simulink model "Richero280245_Assign2"  (R2024b)
settings: Solver=ode5  StartTime=0.0  StopTime=simTime  FixedStep=fixedStepSize  RelTol=1e-3
settings Model: Creator=carlorichero  LastModifiedBy=carlorichero
settings OptimizationCC: DefaultParameterBehavior=Inlined  EnhancedBackFolding=on  PassReuseOutputArgsAs=Individual arguments  ZeroExternalMemoryAtStartup=off  ZeroInternalMemoryAtStartup=off  OptimizeBlockOrder=speed  DifferentSizesBufferReuse=on  OptimizationCustomize=off  EfficientTunableParamExpr=on
settings DebuggingCC: ParameterTunabilityLossMsg=error  ModelReferenceSymbolNameMessage=none
settings ModelReferenceCC: ModelReferenceMinAlgLoopOccurrences=on
settings SFSimCC: MATLABDynamicMemAlloc=off
settings RTWCC: Description=Embedded Coder  SystemTargetFile=ert.tlc  TemplateMakefile=ert_default_tmf
settings CodeAppCC: ForceParamTrailComments=on  IgnoreCustomStorageClasses=off  OperatorAnnotations=on  SimulinkDataObjDesc=on  SFDataObjDesc=on  InsertBlockDesc=on
settings ERTTargetCC: TargetLangStandard=C99 (ISO)  GenerateSampleERTMain=on  SupportContinuousTime=on  ERTCustomFileTemplate=example_file_process.tlc

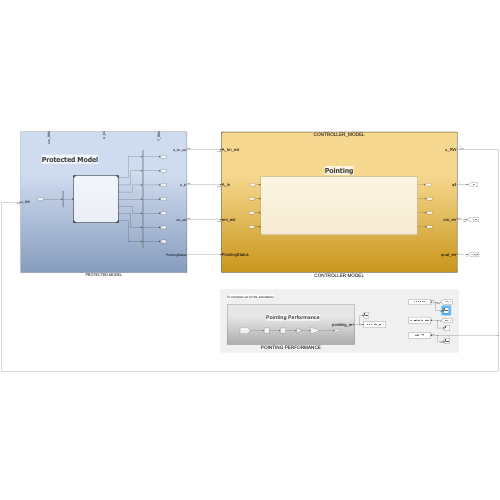
[thumbnail: Simulink's stored preview of the top-level diagram]
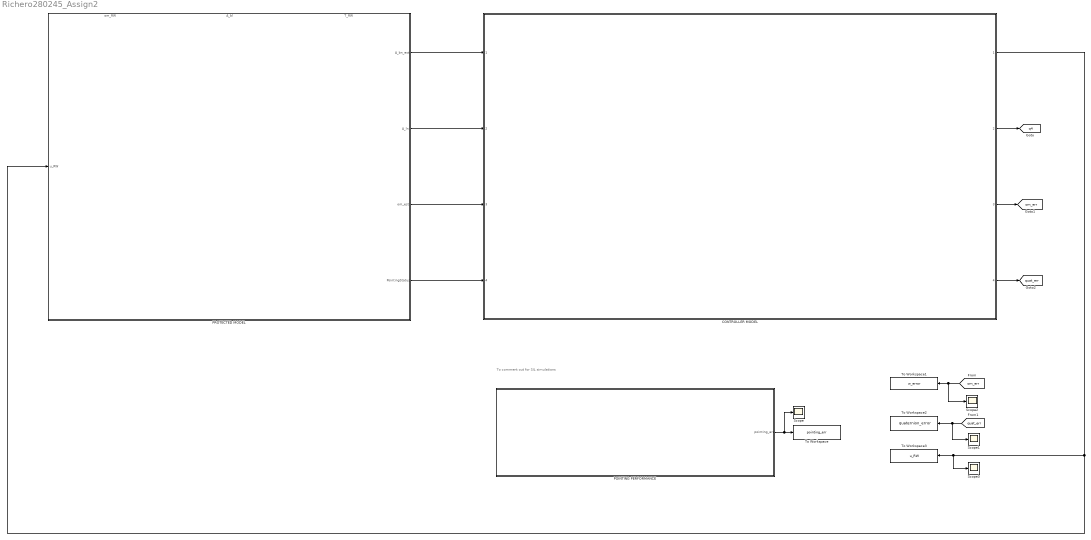
== system Richero280245_Assign2 ==
  note: To comment out for SIL simulations
  CONTROLLER MODEL : Subsystem  TreatAsAtomicUnit=on  ReferencedSubsystem=CONTROLLER_MODEL
  POINTING PERFORMANCE : Subsystem
  PROTECTED MODEL : Subsystem
      settings: PortSchema="{\"entries\":[{\"content\":{\"sides\":[{\"content\":{\"connectorIds\":[\"In1\"]},\"type\":\"ConnectorPlacement.EquallySpacedRectSide\",\"uuid\":\"4269bbd7-3d48-41c9-baab-2de509ebb7e1\"},{\"content\":{\"connectorIds\":[\"Out1\",\"Out2\",\"Out3\",\"Out4\"],\"side\":\"RIGHT\"},\"type\":\"ConnectorPlacement.EquallySpacedRectSide\",\"uuid\":\"222d9627-51e2-4221-8804-06875370038a\"},{\"content\":{\"connectorIds\":[\"Out5\",\"Out6\",\"Out7\"],\"side\":\"TOP\"},\"type\":\"ConnectorPlacement.EquallySpacedRectSide\",\"uuid\":\"776906b1-e520-453d-82b9-997892025e37\"}]},\"type\":\"ConnectorPlacement.EquallySpacedConnector\",\"uuid\":\"d946510d-fad0-4a3e-8089-90c78bf4e7fd\"}],\"packageUris\":[\"http://schema.mathworks.com/mf0/Connector/R2020b\"],\"version\":\"1.0\"}"
  Scope{,1..3} (4 alike) : Scope
  To Workspace : ToWorkspace  VariableName=pointing_err  SampleTime=-1
      settings: Save2DSignal=2-D array (concatenate along first dimension)
  To Workspace1 : ToWorkspace  VariableName=w_error  SampleTime=-1
  To Workspace2 : ToWorkspace  VariableName=quaternion_error  SampleTime=-1
  To Workspace3 : ToWorkspace  VariableName=u_RW  SampleTime=-1
  tag scope: om_err=global, q4=global, quat_err=global
  wires:
  CONTROLLER MODEL/1 -> PROTECTED MODEL/1(u_RW), Scope3/1, To Workspace3/1
  CONTROLLER MODEL/2 -> [q4]
  PROTECTED MODEL/1(A_bn_est) -> CONTROLLER MODEL/1
  PROTECTED MODEL/2(A_ln) -> CONTROLLER MODEL/2
  PROTECTED MODEL/3(om_est) -> CONTROLLER MODEL/3
  PROTECTED MODEL/4(PointingStatus) -> CONTROLLER MODEL/4
  CONTROLLER MODEL/3 -> [om_err]
  CONTROLLER MODEL/4 -> [quat_err]
  POINTING PERFORMANCE/1(pointing_err) -> Scope/1, To Workspace/1
  [quat_err] -> Scope1/1, To Workspace2/1
  [om_err] -> Scope2/1, To Workspace1/1

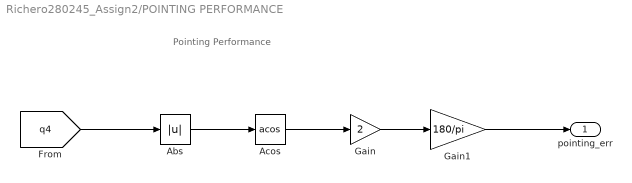
== system Richero280245_Assign2/POINTING PERFORMANCE ==
  note: Pointing Performance
  Abs : Abs  SaturateOnIntegerOverflow=off
  Acos : Trigonometry  Operator=acos
  Gain : Gain  Gain=2
  Gain1 : Gain  Gain=180/pi
  pointing_err : Outport
  wires:
  Acos/1 -> Gain/1
  Abs/1 -> Acos/1
  Gain1/1 -> pointing_err/1
  [q4] -> Abs/1
  Gain/1 -> Gain1/1

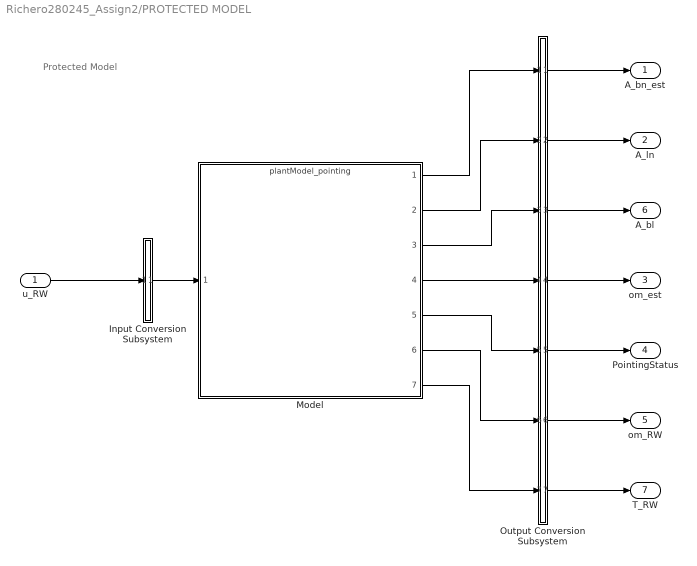
== system Richero280245_Assign2/PROTECTED MODEL ==
  note: Protected Model
  u_RW : Inport
  Input Conversion Subsystem : Subsystem  Tag=__SLT_ICS__  Description=|
      | Signal spec.
      | and routing
      settings: AttributesFormatString=%<Description>
  Model : ModelReference  ModelNameDialog=plantModel_pointing.slxp  ModelReferenceVersion=1.73  CopyOfModelProtected=on
  Output Conversion Subsystem : Subsystem  Tag=__SLT_OCS__  Description=|
      | Signal spec.
      | and routing
      settings: AttributesFormatString=%<Description>
  A_bn_est : Outport
  A_ln : Outport  Port=2
  om_est : Outport  Port=3
  PointingStatus : Outport  Port=4
  om_RW : Outport  Port=5
  A_bl : Outport  Port=6
  T_RW : Outport  Port=7
  wires:
  Model/6 -> Output Conversion Subsystem/6(Inport_6)
  Output Conversion Subsystem/1(Outport_1) -> A_bn_est/1
  Model/2 -> Output Conversion Subsystem/2(Inport_2)
  Output Conversion Subsystem/5(Outport_5) -> PointingStatus/1
  Output Conversion Subsystem/2(Outport_2) -> A_ln/1
  Model/7 -> Output Conversion Subsystem/7(Inport_7)
  Output Conversion Subsystem/7(Outport_7) -> T_RW/1
  Model/1 -> Output Conversion Subsystem/1(Inport_1)
  Model/3 -> Output Conversion Subsystem/3(Inport_3)
  Input Conversion Subsystem/1(Outport_1) -> Model/1
  Model/5 -> Output Conversion Subsystem/5(Inport_5)
  Model/4 -> Output Conversion Subsystem/4(Inport_4)
  Output Conversion Subsystem/6(Outport_6) -> om_RW/1
  Output Conversion Subsystem/4(Outport_4) -> om_est/1
  Output Conversion Subsystem/3(Outport_3) -> A_bl/1
  u_RW/1 -> Input Conversion Subsystem/1(Inport_1)

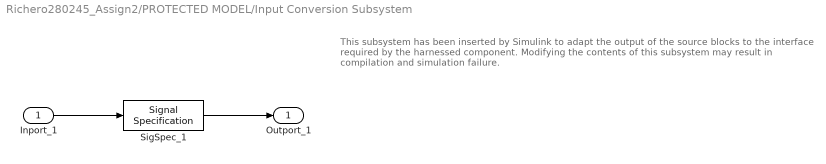
== system Richero280245_Assign2/PROTECTED MODEL/Input Conversion Subsystem ==
  note: This subsystem has been inserted by Simulink to adapt the output of the source blocks to the interface required by the harnessed component.
      |  Modifying the contents of this subsystem may result in compilation and simulation failure.
  Inport_1 : Inport
  SigSpec_1 : SignalSpecification  OutDataTypeStr=double  Dimensions=[3, 1]  SampleTime=0.1
  Outport_1 : Outport
  wires:
  SigSpec_1/1 -> Outport_1/1
  Inport_1/1 -> SigSpec_1/1

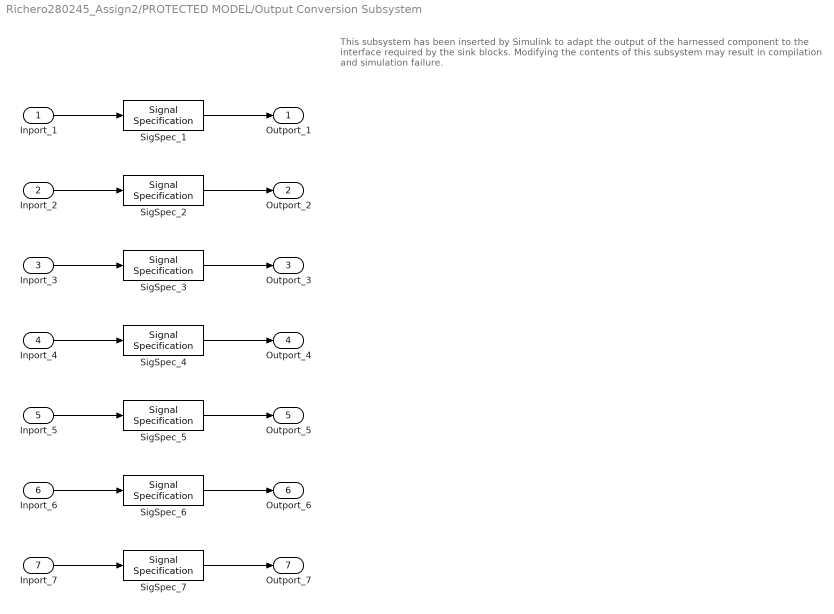
== system Richero280245_Assign2/PROTECTED MODEL/Output Conversion Subsystem ==
  note: This subsystem has been inserted by Simulink to adapt the output of the harnessed component to the interface required by the sink blocks.
      |  Modifying the contents of this subsystem may result in compilation and simulation failure.
  Inport_1 : Inport
  Inport_2 : Inport  Port=2
  Inport_3 : Inport  Port=3
  Inport_4 : Inport  Port=4
  Inport_5 : Inport  Port=5
  Inport_6 : Inport  Port=6
  Inport_7 : Inport  Port=7
  SigSpec_1 : SignalSpecification  OutDataTypeStr=double  Dimensions=[3, 3]
  SigSpec_2 : SignalSpecification  OutDataTypeStr=double  Dimensions=[3, 3]
  SigSpec_3 : SignalSpecification  OutDataTypeStr=double  Dimensions=[3, 3]
  SigSpec_4 : SignalSpecification  OutDataTypeStr=double  Dimensions=[3, 1]
  SigSpec_5 : SignalSpecification  OutDataTypeStr=int32  Dimensions=[1]  SampleTime=0.1
  SigSpec_6 : SignalSpecification  OutDataTypeStr=double  Dimensions=[3, 1]
  SigSpec_7 : SignalSpecification  OutDataTypeStr=double  Dimensions=[3]
  Outport_1 : Outport
  Outport_2 : Outport  Port=2
  Outport_3 : Outport  Port=3
  Outport_4 : Outport  Port=4
  Outport_5 : Outport  Port=5
  Outport_6 : Outport  Port=6
  Outport_7 : Outport  Port=7
  wires:
  Inport_1/1 -> SigSpec_1/1
  SigSpec_1/1 -> Outport_1/1
  Inport_2/1 -> SigSpec_2/1
  SigSpec_2/1 -> Outport_2/1
  Inport_3/1 -> SigSpec_3/1
  SigSpec_3/1 -> Outport_3/1
  Inport_4/1 -> SigSpec_4/1
  SigSpec_4/1 -> Outport_4/1
  Inport_5/1 -> SigSpec_5/1
  SigSpec_5/1 -> Outport_5/1
  Inport_6/1 -> SigSpec_6/1
  SigSpec_6/1 -> Outport_6/1
  Inport_7/1 -> SigSpec_7/1
  SigSpec_7/1 -> Outport_7/1
